simulink model "SSI_model"  (R2017a)
settings: Solver=VariableStepAuto  StartTime=0.0  StopTime=9.9  RelTol=1e-3
values from neighbouring files (symbols this model uses):
  A = double(subs(A_sym, phi_sym, 0))    [create_constants.m]    (also in forward_kinematic_linear.m = [0.7689, 0.0639, -0.1471, 0.0592; linearize_model.m = -1*((Rt / k_m * Z)\(Rt / k_m * V + EM * eye(4,4))); sim_system.m; test.m = [cos(phi), -sin(phi), 0)
  B = double(subs(B_sym, phi_sym, 0))    [create_constants.m]    (also in forward_kinematic_linear.m = [6.8984, -1.9066, 4.3907, -1.7678; linearize_model.m = pinv(Rt / k_m * Z); sim_system.m; test.m = [m, 0, 0)
  BotToWheel = G' / r    [create_constants.m]    (also in find_body_to_wheel_alpha.m = (-1 * G / r)'; graph_max_robot_speeds.m; sim_system.m; test_kalman_filter_LQI.m = -1 * G' / r)
  C = eye(4,4)    [create_constants.m]    (also in sim_system.m; test.m = simplify(C); test_kalman_filter_LQI.m; test_kalman_filter_LQR.m)
  D = zeros(4,4)    [create_constants.m]    (also in sim_system.m; test.m = pinv(G); test_kalman_filter_LQI.m; test_kalman_filter_LQR.m)
  delay = 100    [create_constants.m]
  delay_est = delay * 1    (= 100)    [create_constants.m]
  K2 = K_int(:, 5:8)    [create_constants.m]    (also in sim_system.m; test_kalman_filter_LQI.m = K_int(:, 5:8)*0)
  td = 0    [create_constants.m]    (also in sim_system.m)
  ti = 0    [create_constants.m]    (also in sim_system.m)
  tp = 0    [create_constants.m]    (also in sim_system.m = 2)
  w_n = 1/10    (= 0.1)    [create_constants.m]
  wd = 0    [create_constants.m]    (also in sim_system.m)
  WheelToBot = pinv(BotToWheel)    [create_constants.m]    (also in graph_max_robot_speeds.m; sim_system.m; test_kalman_filter_LQI.m; test_kalman_filter_LQR.m)
  wi = 0    [create_constants.m]    (also in sim_system.m = 0.5)
  wp = 0    [create_constants.m]    (also in sim_system.m = 1)
  X_0 = [0, 0, 0, 0]    [create_constants.m]
undefined symbols (not defined in the file or in its folder): K
libraries: simulink x4
settings Model: Creator=Joe  LastModifiedBy=Joe

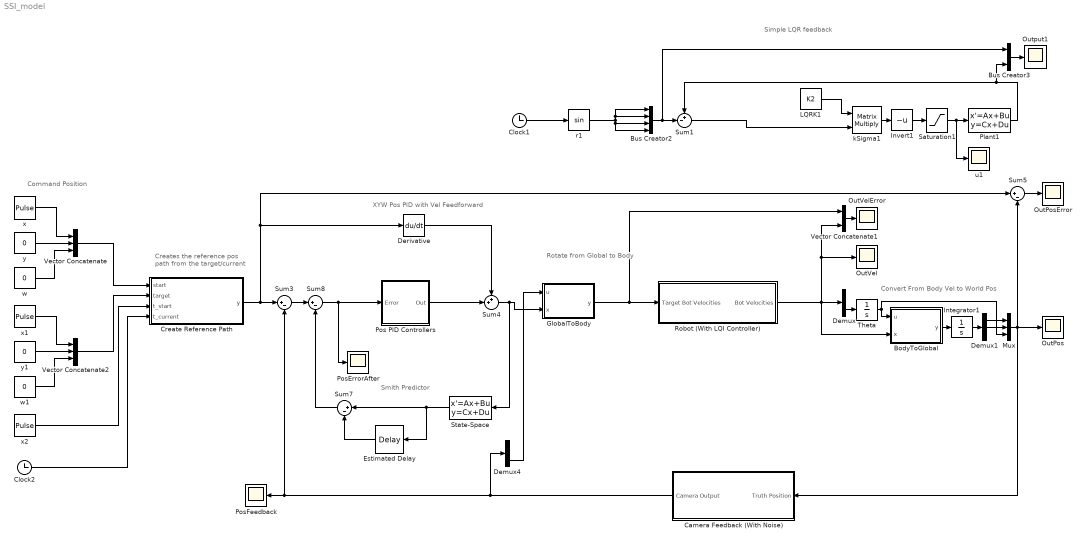
== system SSI_model ==
  note: Smith Predictor
  note: Simple LQR feedback
  note: Creates the reference pos
      | path from the target/current
  note: Rotate from
      | Global to Body
  note: XYW Pos PID with Vel Feedforward
  note: Convert From Body Vel to World Pos
  note: Command Position
  BodyToGlobal : MATLAB Function  TreatAsAtomicUnit=on
  Bus Creator2 : BusCreator  Inputs=4
  Bus Creator3 : BusCreator  Inputs=2
  Camera Feedback (With Noise) : Subsystem
  Clock1 : Clock
  Clock2 : Clock
  Create Reference Path : MATLAB Function  TreatAsAtomicUnit=on
  Demux : Demux  Outputs=3
  Demux1 : Demux  Outputs=3
  Demux4 : Demux  Outputs=3
  Derivative : Derivative
  Estimated Delay : TransportDelay  DelayTime=delay_est
  GlobalToBody : MATLAB Function  TreatAsAtomicUnit=on
  Integrator1 : Integrator
  Invert1 : UnaryMinus
  LQRK1 : Constant  Value=K2
  Mux : Mux  Inputs=3
  OutPos : Scope
  OutPosError : Scope
  OutVel : Scope
  OutVelError : Scope
  Output1 : Scope
  Plant1 : StateSpace  A=A  B=B  C=C  D=D  X0=X_0
  Pos PID Controllers : Subsystem
  PosErrorAfter : Scope
  PosFeedback : Scope
  Robot (With LQI Controller) : Subsystem
  Saturation1 : Saturate  UpperLimit=12  LowerLimit=-12
  State-Space : StateSpace  A=[0,0,0;0,0,0;0,0,0]  B=[1,0,0; 0,1,0; 0,0,1]  C=[1,0,0; 0,1,0; 0,0,1]  D=[0,0,0;0,0,0;0,0,0]  X0=0
  Sum1 : Sum  Inputs=+-|
  Sum{3,5,7..8} (4 alike) : Sum  Inputs=|+-
  Sum4 : Sum  Inputs=++|
  Theta : Integrator
  Vector Concatenate : Concatenate  NumInputs=3
  Vector Concatenate1 : Concatenate
  Vector Concatenate2 : Concatenate  NumInputs=3
  kSigma1 : Product  Multiplication=Matrix(*)
  r1 : Trigonometry
  u1 : Scope
  w : Constant  Value=0
  w1 : Constant  Value=0
  x : DiscretePulseGenerator  PulseType=Time based  Period=10  PulseWidth=50  PhaseDelay=5
  x1 : DiscretePulseGenerator  PulseType=Time based  Period=10  PulseWidth=50
  x2 : DiscretePulseGenerator  PulseType=Time based  Amplitude=5  Period=20  PulseWidth=50  PhaseDelay=5
  y : Constant  Value=0
  y1 : Constant  Value=0
  wires:
  kSigma1/1 -> Invert1/1
  Bus Creator2/1 -> Bus Creator3/1, Sum1/2
  r1/1 -> Bus Creator2/2, Bus Creator2/1, Bus Creator2/3, Bus Creator2/4
  Plant1/1 -> Bus Creator3/2, Sum1/1
  Sum1/1 -> kSigma1/2
  LQRK1/1 -> kSigma1/1
  Invert1/1 -> Saturation1/1
  Bus Creator3/1 -> Output1/1
  Saturation1/1 -> u1/1, Plant1/1
  Clock1/1 -> r1/1
  Vector Concatenate1/1 -> OutVelError/1
  Theta/1 -> BodyToGlobal/1(u), Mux/3
  Demux/3 -> Theta/1
  Demux1/2 -> Mux/2
  Demux1/1 -> Mux/1
  BodyToGlobal/1(y) -> Integrator1/1
  Integrator1/1 -> Demux1/1
  Mux/1 -> Camera Feedback (With Noise)/1(Truth Position), OutPos/1, Sum5/2
  y/1 -> Vector Concatenate/2
  w/1 -> Vector Concatenate/3
  x/1 -> Vector Concatenate/1
  Vector Concatenate/1 -> Create Reference Path/1(start)
  x1/1 -> Vector Concatenate2/1
  y1/1 -> Vector Concatenate2/2
  w1/1 -> Vector Concatenate2/3
  Vector Concatenate2/1 -> Create Reference Path/2(target)
  x2/1 -> Create Reference Path/3(t_start)
  Clock2/1 -> Create Reference Path/4(t_current)
  Create Reference Path/1(y) -> Sum5/1, Derivative/1, Sum3/1
  Derivative/1 -> Sum4/1
  Sum5/1 -> OutPosError/1
  Sum4/1 -> State-Space/1, GlobalToBody/2(x)
  Demux4/3 -> GlobalToBody/1(u)
  Estimated Delay/1 -> Sum7/2
  Sum3/1 -> Sum8/1
  Sum8/1 -> Pos PID Controllers/1(Error), PosErrorAfter/1
  Sum7/1 -> Sum8/2
  State-Space/1 -> Estimated Delay/1, Sum7/1
  Robot (With LQI Controller)/1(Bot Velocities) -> Vector Concatenate1/2, OutVel/1, BodyToGlobal/2(x), Demux/1
  GlobalToBody/1(y) -> Vector Concatenate1/1, Robot (With LQI Controller)/1(Target Bot Velocities)
  Camera Feedback (With Noise)/1(Camera Output) -> Sum3/2, PosFeedback/1, Demux4/1
  Pos PID Controllers/1(Out) -> Sum4/2

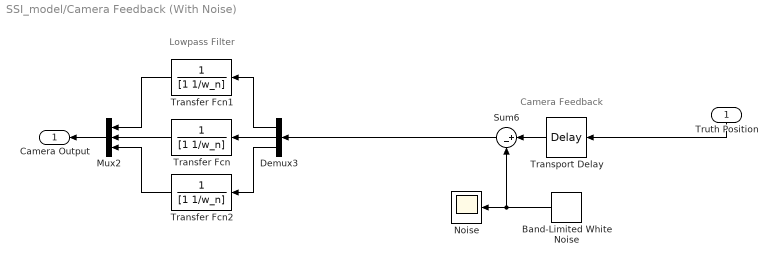
== system SSI_model/Camera Feedback (With Noise) ==
  note: Lowpass Filter
  note: Camera Feedback
  Truth Position : Inport
  Band-Limited White Noise : simulink/Sources/Band-Limited White Noise  Cov=0.00001  Ts=0.01  seed=[23341]
  Demux3 : Demux  Outputs=3
  Mux2 : Mux  Inputs=3
  Noise : Scope
  Sum6 : Sum  Inputs=|+-
  Transfer Fcn : TransferFcn  Denominator=[1 1/w_n]
  Transfer Fcn1 : TransferFcn  Denominator=[1 1/w_n]
  Transfer Fcn2 : TransferFcn  Denominator=[1 1/w_n]
  Transport Delay : TransportDelay  DelayTime=delay
  Camera Output : Outport
  wires:
  Truth Position/1 -> Transport Delay/1
  Transport Delay/1 -> Sum6/1
  Demux3/2 -> Transfer Fcn/1
  Band-Limited White Noise/1 -> Noise/1, Sum6/2
  Demux3/1 -> Transfer Fcn1/1
  Transfer Fcn/1 -> Mux2/2
  Mux2/1 -> Camera Output/1
  Transfer Fcn2/1 -> Mux2/3
  Sum6/1 -> Demux3/1
  Demux3/3 -> Transfer Fcn2/1
  Transfer Fcn1/1 -> Mux2/1

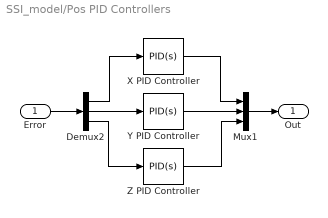
== system SSI_model/Pos PID Controllers ==
  Error : Inport
  Demux2 : Demux  Outputs=3
  Mux1 : Mux  Inputs=3
  X PID Controller : simulink/Continuous/PID Controller  Controller=PID  TimeDomain=Continuous-time  SampleTime=-1  IntegratorMethod=Forward Euler  FilterMethod=Forward Euler  Form=Parallel  UseFilter=on  ControllerParametersSource=internal  P=tp  I=ti  D=td  N=0  InitialConditionSource=internal  InitialConditionForIntegrator=0  InitialConditionForFilter=0  ExternalReset=none  LimitOutput=off  UpperSaturationLimit=inf  LowerSaturationLimit=-inf  LinearizeAsGain=on  AntiWindupMode=none  Kb=1  TrackingMode=off  Kt=1  PParamMin=[]  PParamMax=[]  IParamMin=[]  IParamMax=[]  DParamMin=[]  DParamMax=[]  NParamMin=[]  NParamMax=[]  KbParamMin=[]  KbParamMax=[]  KtParamMin=[]  KtParamMax=[]  POutMin=[]  POutMax=[]  IOutMin=[]  IOutMax=[]  DOutMin=[]  DOutMax=[]  NOutMin=[]  NOutMax=[]  KbOutMin=[]  KbOutMax=[]  KtOutMin=[]  KtOutMax=[]  IntegratorOutMin=[]  IntegratorOutMax=[]  FilterOutMin=[]  FilterOutMax=[]  SumOutMin=[]  SumOutMax=[]  SumI1OutMin=[]  SumI1OutMax=[]  SumI2OutMin=[]  SumI2OutMax=[]  SumI3OutMin=[]  SumI3OutMax=[]  SumDOutMin=[]  SumDOutMax=[]  SaturationOutMin=[]  SaturationOutMax=[]  IntegratorContinuousStateAttributes=''  IntegratorStateMustResolveToSignalObject=off  IntegratorRTWStateStorageClass=Auto  FilterContinuousStateAttributes=''  FilterStateMustResolveToSignalObject=off  FilterRTWStateStorageClass=Auto  DifferentiatorICPrevScaledInput=0  DifferentiatorOutMin=[]  DifferentiatorOutMax=[]  InitialConditionSetting=State (most efficient)
  Y PID Controller : simulink/Continuous/PID Controller  Controller=PID  TimeDomain=Continuous-time  SampleTime=-1  IntegratorMethod=Forward Euler  FilterMethod=Forward Euler  Form=Parallel  UseFilter=on  ControllerParametersSource=internal  P=tp  I=ti  D=td  N=0  InitialConditionSource=internal  InitialConditionForIntegrator=0  InitialConditionForFilter=0  ExternalReset=none  LimitOutput=off  UpperSaturationLimit=inf  LowerSaturationLimit=-inf  LinearizeAsGain=on  AntiWindupMode=none  Kb=1  TrackingMode=off  Kt=1  PParamMin=[]  PParamMax=[]  IParamMin=[]  IParamMax=[]  DParamMin=[]  DParamMax=[]  NParamMin=[]  NParamMax=[]  KbParamMin=[]  KbParamMax=[]  KtParamMin=[]  KtParamMax=[]  POutMin=[]  POutMax=[]  IOutMin=[]  IOutMax=[]  DOutMin=[]  DOutMax=[]  NOutMin=[]  NOutMax=[]  KbOutMin=[]  KbOutMax=[]  KtOutMin=[]  KtOutMax=[]  IntegratorOutMin=[]  IntegratorOutMax=[]  FilterOutMin=[]  FilterOutMax=[]  SumOutMin=[]  SumOutMax=[]  SumI1OutMin=[]  SumI1OutMax=[]  SumI2OutMin=[]  SumI2OutMax=[]  SumI3OutMin=[]  SumI3OutMax=[]  SumDOutMin=[]  SumDOutMax=[]  SaturationOutMin=[]  SaturationOutMax=[]  IntegratorContinuousStateAttributes=''  IntegratorStateMustResolveToSignalObject=off  IntegratorRTWStateStorageClass=Auto  FilterContinuousStateAttributes=''  FilterStateMustResolveToSignalObject=off  FilterRTWStateStorageClass=Auto  DifferentiatorICPrevScaledInput=0  DifferentiatorOutMin=[]  DifferentiatorOutMax=[]  InitialConditionSetting=State (most efficient)
  Z PID Controller : simulink/Continuous/PID Controller  Controller=PID  TimeDomain=Continuous-time  SampleTime=-1  IntegratorMethod=Forward Euler  FilterMethod=Forward Euler  Form=Parallel  UseFilter=on  ControllerParametersSource=internal  P=wp  I=wi  D=wd  N=26080.4758865559  InitialConditionSource=internal  InitialConditionForIntegrator=0  InitialConditionForFilter=0  ExternalReset=none  LimitOutput=off  UpperSaturationLimit=inf  LowerSaturationLimit=-inf  LinearizeAsGain=on  AntiWindupMode=none  Kb=1  TrackingMode=off  Kt=1  PParamMin=[]  PParamMax=[]  IParamMin=[]  IParamMax=[]  DParamMin=[]  DParamMax=[]  NParamMin=[]  NParamMax=[]  KbParamMin=[]  KbParamMax=[]  KtParamMin=[]  KtParamMax=[]  POutMin=[]  POutMax=[]  IOutMin=[]  IOutMax=[]  DOutMin=[]  DOutMax=[]  NOutMin=[]  NOutMax=[]  KbOutMin=[]  KbOutMax=[]  KtOutMin=[]  KtOutMax=[]  IntegratorOutMin=[]  IntegratorOutMax=[]  FilterOutMin=[]  FilterOutMax=[]  SumOutMin=[]  SumOutMax=[]  SumI1OutMin=[]  SumI1OutMax=[]  SumI2OutMin=[]  SumI2OutMax=[]  SumI3OutMin=[]  SumI3OutMax=[]  SumDOutMin=[]  SumDOutMax=[]  SaturationOutMin=[]  SaturationOutMax=[]  IntegratorContinuousStateAttributes=''  IntegratorStateMustResolveToSignalObject=off  IntegratorRTWStateStorageClass=Auto  FilterContinuousStateAttributes=''  FilterStateMustResolveToSignalObject=off  FilterRTWStateStorageClass=Auto  DifferentiatorICPrevScaledInput=0  DifferentiatorOutMin=[]  DifferentiatorOutMax=[]  InitialConditionSetting=State (most efficient)
  Out : Outport
  wires:
  Error/1 -> Demux2/1
  Mux1/1 -> Out/1
  X PID Controller/1 -> Mux1/1
  Demux2/2 -> Y PID Controller/1
  Z PID Controller/1 -> Mux1/3
  Demux2/1 -> X PID Controller/1
  Y PID Controller/1 -> Mux1/2
  Demux2/3 -> Z PID Controller/1

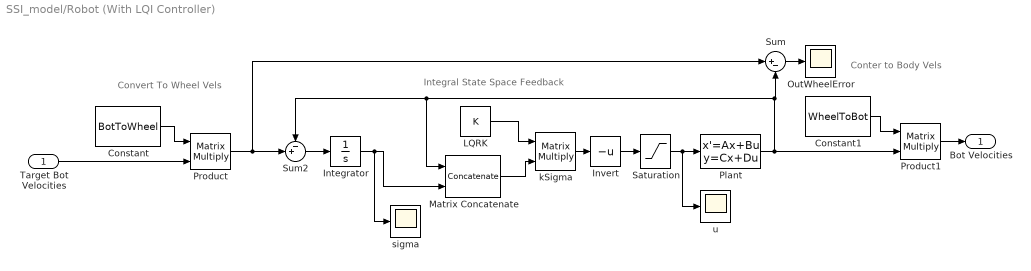
== system SSI_model/Robot (With LQI Controller) ==
  note: Conter to Body Vels
  note: Convert To Wheel Vels
  note: Integral State Space Feedback
  Target Bot Velocities : Inport
  Constant : Constant  Value=BotToWheel
  Constant1 : Constant  Value=WheelToBot
  Integrator : Integrator
  Invert : UnaryMinus
  LQRK : Constant  Value=K
  Matrix Concatenate : Concatenate
  OutWheelError : Scope
  Plant : StateSpace  A=A  B=B  C=C  D=D  X0=X_0
  Product : Product  Multiplication=Matrix(*)
  Product1 : Product  Multiplication=Matrix(*)
  Saturation : Saturate  UpperLimit=12  LowerLimit=-12
  Sum : Sum  Inputs=|+-
  Sum2 : Sum  Inputs=-+|
  kSigma : Product  Multiplication=Matrix(*)
  sigma : Scope
  u : Scope
  Bot Velocities : Outport
  wires:
  Integrator/1 -> sigma/1, Matrix Concatenate/2
  kSigma/1 -> Invert/1
  Saturation/1 -> u/1, Plant/1
  Constant/1 -> Product/1
  LQRK/1 -> kSigma/1
  Constant1/1 -> Product1/1
  Plant/1 -> Product1/2, Matrix Concatenate/1, Sum2/1, Sum/2
  Product/1 -> Sum/1, Sum2/2
  Product1/1 -> Bot Velocities/1
  Sum2/1 -> Integrator/1
  Matrix Concatenate/1 -> kSigma/2
  Invert/1 -> Saturation/1
  Sum/1 -> OutWheelError/1
  Target Bot Velocities/1 -> Product/2

== matlab function SSI_model/Create Reference Path ==
  data: start input; target input; y output; t_start input; t_current input
function y = Create_Ref(start, target, t_start, t_current)
y = zeros(3,1);
for i = 1:3
    a_c = 2; % Max Accel
    s_c = 1; % Max Speed
    t_a = s_c / a_c;
    
    sign = 2*(target(i) > start(i)) - 1;
    
    t_s = sign*(target(i) - start(i))/s_c - t_a;
    t_end = t_start + t_a + t_s + t_a;

    if (abs(start(i) - target(i)) < 0.01)
        y(i) = 0;
        continue;
    end
    
    if t_current < t_start
        y(i) = start(i);
    elseif t_current < t_start + t_a
        y(i) = start(i) + sign*1/2*a_c*(t_current - t_start)^2;
    elseif t_current < t_end - t_a
        y(i) = 1/2*(start(i) + target(i)) + sign*s_c*(t_current - 1/2*(t_start + t_end));
    elseif t_current < t_end
        y(i) = target(i) - sign*1/2*a_c*(t_end - t_current)^2;
    else % t_current > t_end
        y(i) = target(i);
    end
end

== matlab function SSI_model/BodyToGlobal ==
  data: u input; y output; x input
function y =  rotate(u, x)

r = [cos(u), -sin(u), 0;
     sin(u),  cos(u), 0;
          0,       0, 1];
y = r*x;

== matlab function SSI_model/GlobalToBody ==
  data: u input; y output; x input
function y =  rotate(u, x)

r = [cos(u), -sin(u), 0;
     sin(u),  cos(u), 0;
          0,       0, 1];
y = r*x;
